simulink model "simfrecuencia"  (Simulink 7.5)
settings: Solver=ode45  StartTime=0.0  StopTime=10.0  RelTol=1e-3
settings Model: Creator=My Laptop  LastModifiedBy=My Laptop

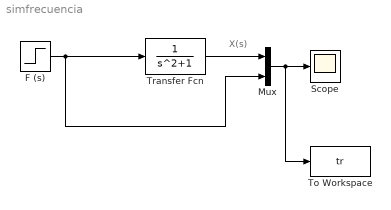
== system simfrecuencia ==
  note: X(s)
  F (s) : Step  SampleTime=0
  Mux : Mux  Inputs=2
  Scope : Scope
      settings: YMin=-1  YMax=1.4
  To Workspace : ToWorkspace  VariableName=tr  SampleTime=-1  SaveFormat=Array
  Transfer Fcn : TransferFcn  Denominator=[1 0 1]
  wires:
  F (s)/1 -> Transfer Fcn/1, Mux/2
  Transfer Fcn/1 -> Mux/1
  Mux/1 -> Scope/1, To Workspace/1
